simulink model "modes_2018b"  (R2018b)
settings: Solver=FixedStepAuto  StartTime=0.0  StopTime=10.0  FixedStep=0.01  RelTol=1e-3  EnableMultiTasking=on
settings Model: ExtModeTrigDuration=5  OrderedModelArguments=off  Creator=junbo  LastModifiedBy=junbo
settings OptimizationCC: DefaultParameterBehavior=Inlined  EnhancedBackFolding=on  PassReuseOutputArgsAs=Individual arguments  MaxStackSize=64  OptimizeBlockOrder=speed  DifferentSizesBufferReuse=on  OptimizationCustomize=off
settings DebuggingCC: ParameterTunabilityLossMsg=error
settings HardwareCC: ProdBitPerPointer=32  ProdBitPerSizeT=32  ProdBitPerPtrDiffT=32  ProdLargestAtomicInteger=Long  ProdLargestAtomicFloat=Double  ProdWordSize=32  ProdHWDeviceType=ARM Compatible->ARM Cortex
settings SFSimCC: MATLABDynamicMemAlloc=off
settings RTWCC: SystemTargetFile=ert.tlc  TemplateMakefile=ert_default_tmf  GenerateReport=on  Toolchain=GNU Tools for ARM Embedded Processors  IncludeHyperlinkInReport=on  LaunchReport=on  GenerateTraceInfo=on  GenerateTraceReport=on  GenerateTraceReportSl=on  GenerateTraceReportSf=on  GenerateTraceReportEml=on
settings CodeAppCC: ForceParamTrailComments=on  IgnoreCustomStorageClasses=off  OperatorAnnotations=on  SimulinkDataObjDesc=on  SFDataObjDesc=on  InsertBlockDesc=on
settings ERTTargetCC: InlinedParameterPlacement=NonHierarchical  ERTCustomFileTemplate=example_file_process.tlc

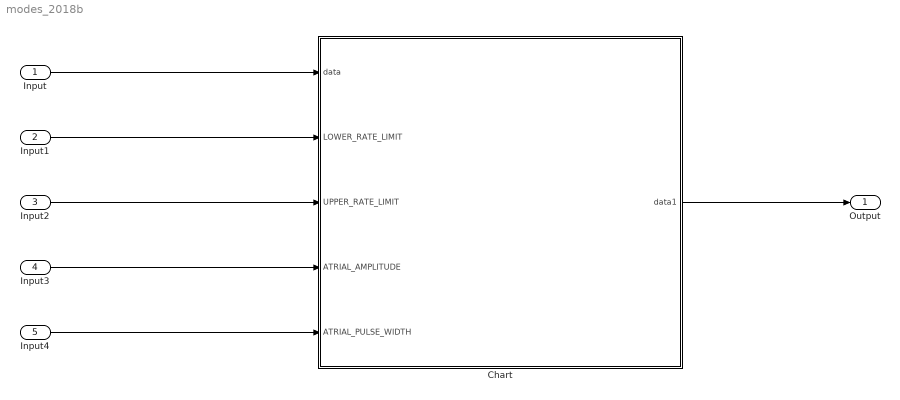
== system modes_2018b ==
  Input : Inport
  Input1 : Inport  Port=2
  Input2 : Inport  Port=3
  Input3 : Inport  Port=4
  Input4 : Inport  Port=5
  Chart : Stateflow chart  TreatAsAtomicUnit=on
  Output : Outport
  wires:
  Input/1 -> Chart/1(data)
  Chart/1(data1) -> Output/1
  Input1/1 -> Chart/2(LOWER_RATE_LIMIT)
  Input2/1 -> Chart/3(UPPER_RATE_LIMIT)
  Input3/1 -> Chart/4(ATRIAL_AMPLITUDE)
  Input4/1 -> Chart/5(ATRIAL_PULSE_WIDTH)

== stateflow chart modes_2018b/Chart ==
  state AOO
  state VOO
  state ChargingState
    entry:
    ATR_PACE_CTRL = false;
    VENT_PACE_CTRL = false;
    PACE_CHARGE_CTRL = true;
  state startState
    entry:
  state AAI
  state VVI
  (junction 14) -> AOO [order 1] : [mode == 1]
  (junction 14) -> VOO [order 2] : [mode == 2]
  ChargingState -> (junction 14)
  (default) -> startState
  startState -> ChargingState
  (junction 14) -> AAI [order 3] : [mode == 3]
  (junction 14) -> VVI [order 4] : [mode == 4]
  data: data input; data1 output; LOWER_RATE_LIMIT input; UPPER_RATE_LIMIT input; ATRIAL_AMPLITUDE input; ATRIAL_PULSE_WIDTH input
